simulink model "bitwiseop_test"  (Simulink 8.4)
settings: Solver=VariableStepDiscrete  StartTime=0.0  StopTime=0  MaxStep=1  RelTol=1e-3
libraries: simulink x9
settings Model: Creator=arnaud  LastModifiedBy=arnaud
settings DataIOCC: SaveFormat=StructureWithTime

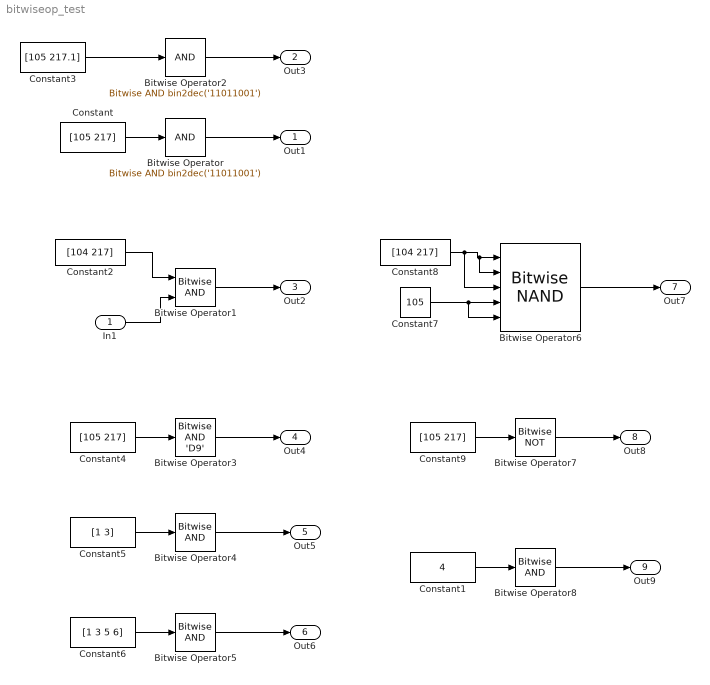
== system bitwiseop_test ==
  In1 : Inport
  Bitwise Operator : simulink/Logic and Bit Operations/Bitwise Operator  logicop=AND  UseBitMask=on  BitMask=bin2dec('11011001')  BitMaskRealWorld=Real World Value
  Bitwise Operator1 : simulink/Logic and Bit Operations/Bitwise Operator  logicop=AND  UseBitMask=off  NumInputPorts=2  BitMask=bin2dec('11011001')  BitMaskRealWorld=Stored Integer
  Bitwise Operator2 : simulink/Logic and Bit Operations/Bitwise Operator  logicop=AND  UseBitMask=on  BitMask=bin2dec('11011001')  BitMaskRealWorld=Stored Integer
  Bitwise Operator3 : simulink/Logic and Bit Operations/Bitwise Operator  logicop=AND  UseBitMask=on  BitMask='D9'  BitMaskRealWorld=Stored Integer
  Bitwise Operator4 : simulink/Logic and Bit Operations/Bitwise Operator  logicop=AND  UseBitMask=off  BitMask=bin2dec('11011001')  BitMaskRealWorld=Real World Value
  Bitwise Operator5 : simulink/Logic and Bit Operations/Bitwise Operator  logicop=AND  UseBitMask=off  BitMask=bin2dec('11011001')  BitMaskRealWorld=Real World Value
  Bitwise Operator6 : simulink/Logic and Bit Operations/Bitwise Operator  logicop=NAND  UseBitMask=off  NumInputPorts=5  BitMask=bin2dec('11011001')  BitMaskRealWorld=Stored Integer
  Bitwise Operator7 : simulink/Logic and Bit Operations/Bitwise Operator  logicop=NOT  UseBitMask=on  BitMask='D9'  BitMaskRealWorld=Stored Integer
  Bitwise Operator8 : simulink/Logic and Bit Operations/Bitwise Operator  logicop=AND  UseBitMask=off  BitMask=bin2dec('11011001')  BitMaskRealWorld=Real World Value
  Constant : Constant  Value=[105 217]  OutDataTypeStr=int32
  Constant1 : Constant  Value=4  OutDataTypeStr=int32
  Constant2 : Constant  Value=[104 217]  OutDataTypeStr=int32
  Constant3 : Constant  Value=[105 217.1]  OutDataTypeStr=fixdt(1,16)
  Constant4 : Constant  Value=[105 217]  OutDataTypeStr=int32
  Constant5 : Constant  Value=[1 3]  OutDataTypeStr=int32
  Constant6 : Constant  Value=[1 3 5 6]  OutDataTypeStr=int32
  Constant7 : Constant  Value=105  OutDataTypeStr=int32
  Constant8 : Constant  Value=[104 217]  OutDataTypeStr=int32
  Constant9 : Constant  Value=[105 217]  OutDataTypeStr=int32
  Out1 : Outport
  Out3 : Outport  Port=2
  Out2 : Outport  Port=3
  Out4 : Outport  Port=4
  Out5 : Outport  Port=5
  Out6 : Outport  Port=6
  Out7 : Outport  Port=7
  Out8 : Outport  Port=8
  Out9 : Outport  Port=9
  wires:
  Bitwise Operator/1 -> Out1/1
  Constant/1 -> Bitwise Operator/1
  Bitwise Operator1/1 -> Out2/1
  In1/1 -> Bitwise Operator1/2
  Constant2/1 -> Bitwise Operator1/1
  Bitwise Operator2/1 -> Out3/1
  Constant3/1 -> Bitwise Operator2/1
  Bitwise Operator3/1 -> Out4/1
  Constant4/1 -> Bitwise Operator3/1
  Bitwise Operator4/1 -> Out5/1
  Constant5/1 -> Bitwise Operator4/1
  Bitwise Operator5/1 -> Out6/1
  Constant6/1 -> Bitwise Operator5/1
  Bitwise Operator6/1 -> Out7/1
  Constant7/1 -> Bitwise Operator6/4, Bitwise Operator6/5
  Constant8/1 -> Bitwise Operator6/3, Bitwise Operator6/2, Bitwise Operator6/1
  Bitwise Operator7/1 -> Out8/1
  Constant9/1 -> Bitwise Operator7/1
  Bitwise Operator8/1 -> Out9/1
  Constant1/1 -> Bitwise Operator8/1
